simulink model "Model_nieliniowy"  (R2017a)
settings: Solver=ode45  StartTime=0.0  StopTime=100  MaxStep=0.1  RelTol=1e-3  EnableMultiTasking=on
values from neighbouring files (symbols this model uses):
  A = pi*R1*R1    (= 10.9999393421)    [Lab2.m]    (also in ModelDataNonlinear.m)
  B = (pi*R2*R2)/(3*H2*H2)    (= 0.00337009933323)    [Lab2.m]    (also in Lab8.m = deltah20max / k; Lab9.m = 0.4; ModelDataNonlinear.m)
  C1 = 1.372    [Lab2.m]    (also in ModelDataNonlinear.m)
  C2 = 0.332756    [Lab2.m]    (also in ModelDataNonlinear.m)
  q10 = C2*sqrt(h20)    [Lab2.m]    (also in ModelDataNonlinear.m)
settings Model: Creator=Ituriello  LastModifiedBy=ishiguro
settings DataIOCC: LimitDataPoints=on  SaveFormat=Array
settings OptimizationCC: LifeSpan=inf
settings DebuggingCC: SFUnexpectedBacktrackingDiag=warning  SFNoUnconditionalDefaultTransitionDiag=warning  SFExecutionAtInitializationDiag=none
settings HardwareCC: ProdBitPerPointer=32  ProdBitPerSizeT=32  ProdBitPerPtrDiffT=32  ProdLargestAtomicFloat=None  ProdIntDivRoundTo=Undefined  ProdEndianess=Unspecified  ProdWordSize=32  ProdHWDeviceType=32-bit Generic
settings ModelReferenceCC: PropagateSignalLabelsOutOfModel=off
settings GRTTargetCC: TargetLangStandard=C89/C90 (ANSI)  GeneratePreprocessorConditionals=Disable all
settings ConfigComp: CovMetricSettings=dw  CovHtmlReporting=on  CovSaveCumulativeToWorkspaceVar=on  CovSaveSingleToWorkspaceVar=on  CovExternalEMLEnable=off

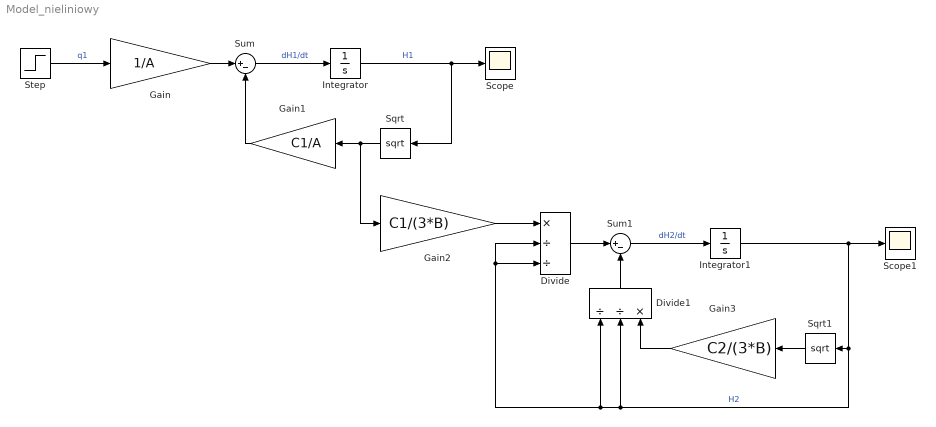
== system Model_nieliniowy ==
  Divide : Product  Inputs=*//
  Divide1 : Product  Inputs=//*
  Gain : Gain  Gain=1/A
  Gain1 : Gain  Gain=C1/A
  Gain2 : Gain  Gain=C1/(3*B)
  Gain3 : Gain  Gain=C2/(3*B)
  Integrator : Integrator
  Integrator1 : Integrator  InitialCondition=4
  Scope : Scope
  Scope1 : Scope
  Sqrt : Sqrt  SaturateOnIntegerOverflow=on
  Sqrt1 : Sqrt  SaturateOnIntegerOverflow=on
  Step : Step  Time=0  After=q10  SampleTime=0
  Sum : Sum  Inputs=|+-
  Sum1 : Sum  Inputs=|+-
  wires:
  Step/1 -> Gain/1  "q1"
  Sum/1 -> Integrator/1  "dH1/dt"
  Integrator/1 -> Sqrt/1, Scope/1  "H1"
  Gain/1 -> Sum/1
  Sqrt/1 -> Gain2/1, Gain1/1
  Gain1/1 -> Sum/2
  Sum1/1 -> Integrator1/1  "dH2/dt"
  Sqrt1/1 -> Gain3/1
  Integrator1/1 -> Scope1/1, Sqrt1/1, Divide1/2, Divide1/1, Divide/3, Divide/2  "H2"
  Gain2/1 -> Divide/1
  Divide/1 -> Sum1/1
  Divide1/1 -> Sum1/2
  Gain3/1 -> Divide1/3
